simulink model "a02_step"  (R2018a)
settings: Solver=VariableStepAuto  StartTime=0.0  StopTime=10.0  RelTol=1e-3
settings Model: Creator=oleksandra  LastModifiedBy=oleksandra

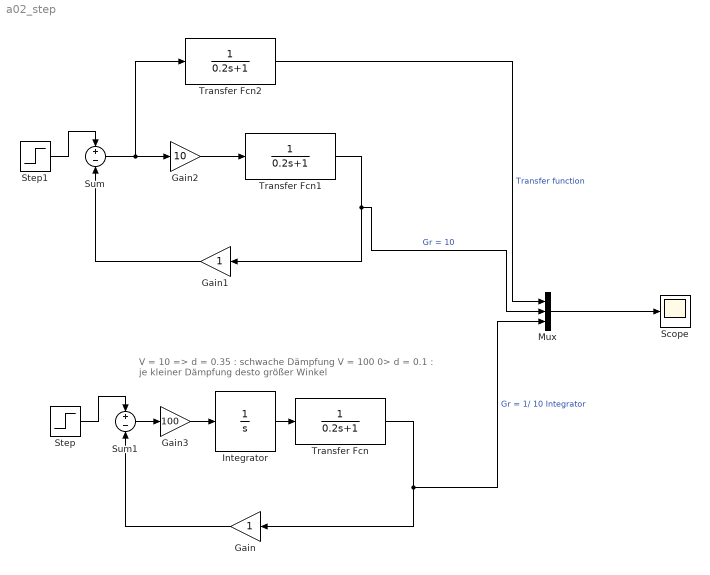
== system a02_step ==
  note: V = 10 => d = 0.35 : schwache Dämpfung
      | V = 100 0> d = 0.1 : je kleiner Dämpfung desto größer Winkel
  Gain : Gain
  Gain1 : Gain
  Gain2 : Gain  Gain=10
  Gain3 : Gain  Gain=100
  Integrator : Integrator
  Mux : Mux  Inputs=3
  Scope : Scope
  Step : Step  SampleTime=0
  Step1 : Step  SampleTime=0
  Sum : Sum  Inputs=+-
  Sum1 : Sum  Inputs=+-
  Transfer Fcn : TransferFcn  Denominator=[0.2 1]
  Transfer Fcn1 : TransferFcn  Denominator=[0.2 1]
  Transfer Fcn2 : TransferFcn  Denominator=[0.2 1]
  wires:
  Sum/1 -> Transfer Fcn2/1, Gain2/1
  Mux/1 -> Scope/1
  Transfer Fcn/1 -> Mux/3, Gain/1  "Gr = 1/ 10 Integrator"
  Integrator/1 -> Transfer Fcn/1
  Step1/1 -> Sum/1
  Gain1/1 -> Sum/2
  Step/1 -> Sum1/1
  Gain/1 -> Sum1/2
  Transfer Fcn1/1 -> Mux/2, Gain1/1  "Gr = 10"
  Gain2/1 -> Transfer Fcn1/1
  Sum1/1 -> Gain3/1
  Gain3/1 -> Integrator/1
  Transfer Fcn2/1 -> Mux/1  "Transfer function"
